simulink library "Backhoe_Lib"  (R2014a)
settings: Solver=ode45  StartTime=0.0  StopTime=10.0  RelTol=1e-3
undefined symbols (not defined in the file): cylinderGray, gcbh, pistonGray, rhoSteel, simmechanics, X, Y, Z
libraries: sm_lib x40, Backhoe_Lib x7, fl_lib x7, nesl_utility x2
(part 2 of 2)

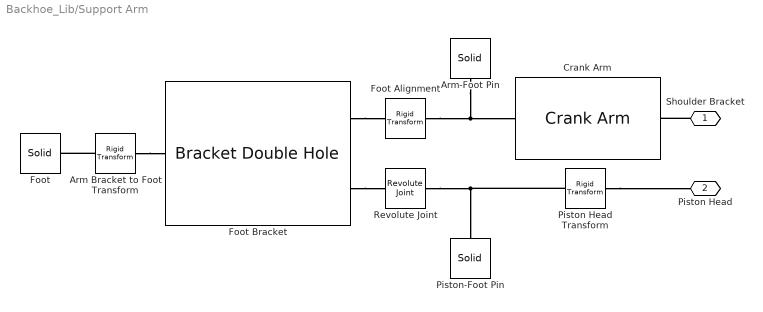
== system Backhoe_Lib/Support Arm ==
  Arm Bracket to Foot Transform : sm_lib/Frames and  Transforms/Rigid  Transform  TranslationMethod=StandardAxis  TranslationLengthUnit=m  TranslationStandardAxis=-Z  TranslationStandardOffset=Tfoot/2  TranslationCartesianOffset=[-Dconn/2 0 -Tfoot/2]  TranslationROffset=0  TranslationROffsetUnits=m  TranslationZOffset=0  TranslationZOffsetUnits=m  TranslationThetaOffset=0  TranslationThetaOffsetUnits=deg  RotationMethod=None  RotationAngleUnits=deg  RotationStandardAxis=-Z  RotationAngle=45  RotationArbitraryAxis=[0 0 1]  FollAlignAxisA=+X  BaseAlignAxisA=+Y  FollAlignAxisB=+Y  BaseAlignAxisB=+Z  BlockFunction=simmechanics.library.frames_transforms.rigid_transform
  Arm-Foot Pin : sm_lib/Body Elements/Solid  InertiaType=CalculateFromGeometry  Mass=1  MassUnits=kg  CenterOfMass=[0 0 0]  CenterOfMassUnits=m  MomentsOfInertia=[1 1 1]  MomentsOfInertiaUnits=kg*m^2  ProductsOfInertia=[0 0 0]  ProductsOfInertiaUnits=kg*m^2  DensityBased=on  Density=rho  DensityUnits=kg/(m^3)  GraphicType=FromGeometry  MarkerShape=Sphere  MarkerSize=10  MarkerSizeUnits=m  GraphicVisPropType=SimpleVisualProperties  GraphicDiffuseColor=pinColor  GraphicSpecularColor=[0.5 0.5 0.5 1.0]  GraphicAmbientColor=[0.15 0.15 0.15 1.0]  GraphicEmissiveColor=[0.0 0.0 0.0 1.0]  GraphicShininess=75  GraphicOpacity=1.0  GeometryShape=Cylinder  RectangleSize=[1 1]  RectangleSizeUnits=m  BrickDimensions=[1 1 1]  BrickDimensionUnits=m  CylinderRadius=Rhole  CylinderRadiusUnits=m  CylinderLength=Lpin  CylinderLengthUnits=m  SphereRadius=1  SphereRadiusUnits=m  EllipsoidRadii=[1 1 1]  EllipsoidRadiiUnits=m  ExtrusionCrossSection=[1 1; 1 1]  ExtrusionCrossSectionUnits=m  ExtrusionLength=Lpin  ExtrusionLengthUnits=m  PolygonNumSides=3  PolygonOuterRadius=1  PolygonOuterRadiusUnits=m  ExtGeomFileUnits=m  RevolutionCrossSection=[1 1; 1 -1; 2 -1; 2 1]  RevolutionCrossSectionUnits=m  RevolutionExtent=Full  RevolutionAngle=180  RevolutionAngleUnits=deg  BlockFunction=simmechanics.library.body_elements.solid
  Crank Arm : Backhoe_Lib/Crank Arm  L=Larm  W=Warm  T=Tarm  D=Dhole  R=Rhole  Nc=25  color=armColor  rho=rho
  Foot : sm_lib/Body Elements/Solid  InertiaType=CalculateFromGeometry  Mass=1  MassUnits=kg  CenterOfMass=[0 0 0]  CenterOfMassUnits=m  MomentsOfInertia=[1 1 1]  MomentsOfInertiaUnits=kg*m^2  ProductsOfInertia=[0 0 0]  ProductsOfInertiaUnits=kg*m^2  DensityBased=on  Density=rho  DensityUnits=kg/(m^3)  GraphicType=FromGeometry  MarkerShape=Sphere  MarkerSize=10  MarkerSizeUnits=m  GraphicVisPropType=SimpleVisualProperties  GraphicDiffuseColor=footColor  GraphicSpecularColor=[0.5 0.5 0.5 1.0]  GraphicAmbientColor=[0.15 0.15 0.15 1.0]  GraphicEmissiveColor=[0.0 0.0 0.0 1.0]  GraphicShininess=75  GraphicOpacity=1.0  GeometryShape=Brick  RectangleSize=[1 1]  RectangleSizeUnits=m  BrickDimensions=[Lfoot Wfoot Tfoot]  BrickDimensionUnits=m  CylinderRadius=1  CylinderRadiusUnits=m  CylinderLength=1  CylinderLengthUnits=m  SphereRadius=1  SphereRadiusUnits=m  EllipsoidRadii=[1 1 1]  EllipsoidRadiiUnits=m  ExtrusionCrossSection=[0 1;1 0; 1 1]  ExtrusionCrossSectionUnits=m  ExtrusionLength=1  ExtrusionLengthUnits=m  PolygonNumSides=3  PolygonOuterRadius=1  PolygonOuterRadiusUnits=m  ExtGeomFileUnits=m  RevolutionCrossSection=[1 1; 1 -1; 2 -1; 2 1]  RevolutionCrossSectionUnits=m  RevolutionExtent=Full  RevolutionAngle=180  RevolutionAngleUnits=deg  BlockFunction=simmechanics.library.body_elements.solid
  Foot Alignment : sm_lib/Frames and  Transforms/Rigid  Transform  TranslationMethod=None  TranslationLengthUnit=m  TranslationStandardAxis=+Z  TranslationStandardOffset=0  TranslationCartesianOffset=[0 0 0]  TranslationROffset=0  TranslationROffsetUnits=m  TranslationZOffset=0  TranslationZOffsetUnits=m  TranslationThetaOffset=0  TranslationThetaOffsetUnits=deg  RotationMethod=StandardAxis  RotationAngleUnits=deg  RotationStandardAxis=+Z  RotationAngle=initAngle  RotationArbitraryAxis=[0 0 1]  FollAlignAxisA=+X  BaseAlignAxisA=+Y  FollAlignAxisB=+Y  BaseAlignAxisB=+Z  BlockFunction=simmechanics.library.frames_transforms.rigid_transform
  Foot Bracket : Backhoe_Lib/Bracket Double Hole  Hbracket=Hhole + Rfillet  Wbracket=Dconn + Rfillet  Tbracket=Tfoot  Dbracket=Wfoot*0.75  Hhole=Hhole  Dhole=Dconn  Rhole=Rhole  Rfillet=Rfillet  Nc=25  bracketColor=bracketColor  rho=rho
  Piston Head Transform : sm_lib/Frames and Transforms/Rigid Transform  TranslationMethod=None  TranslationLengthUnit=m  TranslationStandardAxis=+Z  TranslationStandardOffset=0  TranslationCartesianOffset=[0 0 0]  TranslationROffset=0  TranslationROffsetUnits=m  TranslationZOffset=0  TranslationZOffsetUnits=m  TranslationThetaOffset=0  TranslationThetaOffsetUnits=deg  RotationMethod=AlignedAxes  RotationAngleUnits=deg  RotationStandardAxis=+Z  RotationAngle=0  RotationArbitraryAxis=[0 0 1]  FollAlignAxisA=+Z  BaseAlignAxisA=-Z  FollAlignAxisB=+Y  BaseAlignAxisB=-Y  BlockFunction=simmechanics.library.frames_transforms.rigid_transform
  Piston-Foot Pin : sm_lib/Body Elements/Solid  InertiaType=CalculateFromGeometry  Mass=1  MassUnits=kg  CenterOfMass=[0 0 0]  CenterOfMassUnits=m  MomentsOfInertia=[1 1 1]  MomentsOfInertiaUnits=kg*m^2  ProductsOfInertia=[0 0 0]  ProductsOfInertiaUnits=kg*m^2  DensityBased=on  Density=rho  DensityUnits=kg/(m^3)  GraphicType=FromGeometry  MarkerShape=Sphere  MarkerSize=10  MarkerSizeUnits=m  GraphicVisPropType=SimpleVisualProperties  GraphicDiffuseColor=pinColor  GraphicSpecularColor=[0.5 0.5 0.5 1.0]  GraphicAmbientColor=[0.15 0.15 0.15 1.0]  GraphicEmissiveColor=[0.0 0.0 0.0 1.0]  GraphicShininess=75  GraphicOpacity=1.0  GeometryShape=Cylinder  RectangleSize=[1 1]  RectangleSizeUnits=m  BrickDimensions=[1 1 1]  BrickDimensionUnits=m  CylinderRadius=Rhole  CylinderRadiusUnits=m  CylinderLength=Lpin  CylinderLengthUnits=m  SphereRadius=1  SphereRadiusUnits=m  EllipsoidRadii=[1 1 1]  EllipsoidRadiiUnits=m  ExtrusionCrossSection=[1 1; 1 1]  ExtrusionCrossSectionUnits=m  ExtrusionLength=Lpin  ExtrusionLengthUnits=m  PolygonNumSides=3  PolygonOuterRadius=1  PolygonOuterRadiusUnits=m  ExtGeomFileUnits=m  RevolutionCrossSection=[1 1; 1 -1; 2 -1; 2 1]  RevolutionCrossSectionUnits=m  RevolutionExtent=Full  RevolutionAngle=180  RevolutionAngleUnits=deg  BlockFunction=simmechanics.library.body_elements.solid
  Revolute Joint : sm_lib/Joints/Revolute Joint  SenseConstraintForceX=off  SenseConstraintForceY=off  SenseConstraintForceZ=off  SenseConstraintTorqueX=off  SenseConstraintTorqueY=off  SenseConstraintTorqueZ=off  ConstraintWrenchDir=FollowerOnBase  ConstraintWrenchFrame=BaseFrame  EquilibriumPosition=0  EquilibriumPositionUnits=deg  SpringStiffness=0  SpringStiffnessUnits=N*m/deg  DampingCoefficient=0  DampingCoefficientUnits=N*m/(deg/s)  ActuationMode=NoActuation  SensePosition=off  SenseVelocity=off  SenseAcceleration=off  SenseTorqueForce=off  PositionTargetValue=0  PositionTargetValueUnits=deg  PositionTargetSpecify=off  PositionTargetPriority=High  VelocityTargetValue=0  VelocityTargetValueUnits=deg/s  VelocityTargetSpecify=off  VelocityTargetPriority=High  BlockFunction=simmechanics.library.joints.revolute_joint
  Shoulder Bracket : PMIOPort  Port=1  Side=Right
  Piston Head : PMIOPort  Port=2  Side=Left
  connections:
  Shoulder Bracket/RConn1 -- Crank Arm/RConn1
  Revolute Joint/RConn1 -- Piston Head Transform/LConn1 -- Piston-Foot Pin/RConn1
  Arm Bracket to Foot Transform/RConn1 -- Foot/RConn1
  Arm-Foot Pin/RConn1 -- Crank Arm/LConn1 -- Foot Alignment/RConn1
  Foot Bracket/RConn2 -- Revolute Joint/LConn1
  Foot Bracket/RConn1 -- Foot Alignment/LConn1
  Arm Bracket to Foot Transform/LConn1 -- Foot Bracket/LConn1
  Piston Head Transform/RConn1 -- Piston Head/RConn1

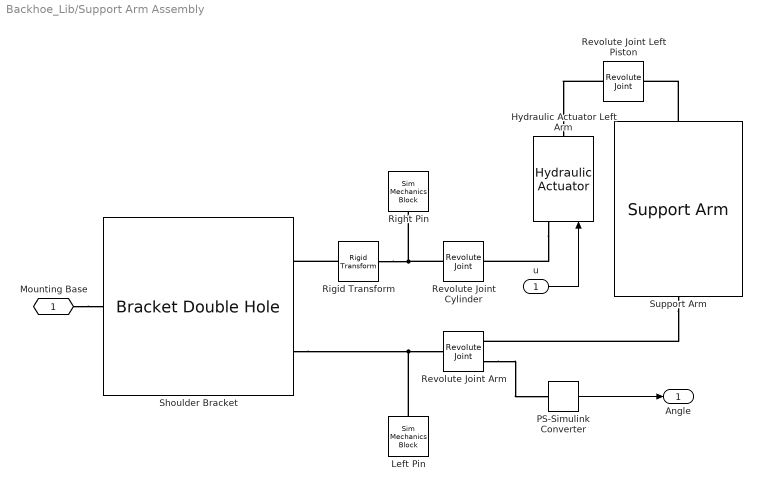
== system Backhoe_Lib/Support Arm Assembly ==
  u : Inport
  Hydraulic Actuator Left Arm : Backhoe_Lib/Hydraulic Actuator  Lcyl=1.35  Rcyl=0.2  Lpist=1.35  Rpist=0.1  Lbase=0.65  Wbase=0.425  Rbp=0.075  Lbp=0.8  Whead=0.275  Lhead=0.5  Rhp=0.075  Lhp=0.9  circlePoints=25  cylColor=cylinderGray  rhoCyl=rho  pistColor=pistonGray  rhoPist=rho  connColor=pinColor  rhoConn=rho
  Left Pin : SimMechanicsBlock  LoadFcn=simmechanics.sli.internal.rtm_callback('LoadFcn',gcbh)  StartFcn=simmechanics.sli.internal.model_callback(bdroot(gcbh),'start');  StopFcn=simmechanics.sli.internal.model_callback(bdroot(gcbh),'stop');  mask(Solid){ClassName=Solid, InertiaType=CalculateFromGeometry, Mass=1, MassUnits=kg, CenterOfMass=[0 0 0], CenterOfMassUnits=m, MomentsOfInertia=[1 1 1], MomentsOfInertiaUnits=kg*m^2, ProductsOfInertia=[0 0 0], ProductsOfInertiaUnits=kg*m^2, DensityBased=on, Density=rho, DensityUnits=kg/(m^3), GraphicType=FromGeometry, MarkerShape=Sphere, MarkerSize=10, MarkerSizeUnits=m, GraphicVisPropType=SimpleVisualProperties, GraphicDiffuseColor=pinColor, GraphicSpecularColor=[0.5 0.5 0.5 1.0], GraphicAmbientColor=[0.15 0.15 0.15 1.0], GraphicEmissiveColor=[0.0 0.0 0.0 1.0], GraphicShininess=75, GraphicOpacity=1.0, GeometryShape=Cylinder, RectangleSize=[1 1], RectangleSizeUnits=m, BrickDimensions=[1 1 1], BrickDimensionUnits=m, CylinderRadius=Rhole, CylinderRadiusUnits=m, CylinderLength=Lpin, CylinderLengthUnits=m, SphereRadius=1, SphereRadiusUnits=m, EllipsoidRadii=[1 1 1], EllipsoidRadiiUnits=m, ExtrusionCrossSection=[1 1; 1 1], ExtrusionCrossSectionUnits=m, ExtrusionLength=1, ExtrusionLengthUnits=m, PolygonNumSides=3, PolygonOuterRadius=1, PolygonOuterRadiusUnits=m, ExtGeomFileName=, ExtGeomFileUnits=m, RevolutionCrossSection=[1 1; 1 -1; 2 -1; 2 1], RevolutionCrossSectionUnits=m, RevolutionExtent=Full, RevolutionAngle=180, RevolutionAngleUnits=deg, BlockFunction=simmechanics.library.body_elements.solid}
      mask prompts: BlockFunction "Block Function"
      settings: PreSaveFcn=simmechanics.sli.internal.rtm_callback('PreSaveFcn',gcbh)  PauseFcn=simmechanics.sli.internal.model_callback(bdroot(gcbh),'pause');  PreCopyFcn=simmechanics.sli.internal.rtm_callback('PreCopyFcn',gcbh)  OpenFcn=simmechanics.sli.internal.block_dialog(gcbh,'open');  CloseFcn=simmechanics.sli.internal.block_dialog(gcbh,'close');  PreDeleteFcn=simmechanics.sli.internal.rtm_callback('PreDeleteFcn',gcbh)
      settings: CopyFcn=|
      | simmechanics.sli.internal.block_dialog(gcbh,'close');
      | simmechanics.sli.internal.rtm_callback('CopyFcn',gcbh)
      settings: DeleteFcn=|
      | simmechanics.sli.internal.block_dialog(gcbh,'close');
      | simmechanics.sli.internal.rtm_callback('DeleteFcn',gcbh)
      settings: ModelCloseFcn=|
      | simmechanics.sli.internal.model_editor_callback(bdroot(gcbh),'close');
      | simmechanics.sli.internal.rtm_callback('ModelCloseFcn',gcbh)
      | simmechanics.sli.internal.model_callback(bdroot(gcbh),'close');
      settings: PostSaveFcn=|
      | simmechanics.sli.internal.model_editor_callback(bdroot(gcbh),'save');
      | simmechanics.sli.internal.rtm_callback('PostSaveFcn',gcbh)
      mask Help: web(simmechanics.sli.internal.block_help(gcbh))
      mask Display: plot([0;1;1;0;0],[0;0;1;1;0]);
  PS-Simulink Converter : nesl_utility/PS-Simulink Converter  PhysicalDomain=network_engine_domain  LeftPortType=input  RightPortType=output  SubClassName=ps_output  PseudoPeriodic=off  Frequencies=[]  Unit=deg  AffineConversion=off
  Revolute Joint Arm : sm_lib/Joints/Revolute Joint  SenseConstraintForceX=off  SenseConstraintForceY=off  SenseConstraintForceZ=off  SenseConstraintTorqueX=off  SenseConstraintTorqueY=off  SenseConstraintTorqueZ=off  ConstraintWrenchDir=FollowerOnBase  ConstraintWrenchFrame=BaseFrame  EquilibriumPosition=0  EquilibriumPositionUnits=deg  SpringStiffness=0  SpringStiffnessUnits=N*m/deg  DampingCoefficient=0  DampingCoefficientUnits=N*m/(deg/s)  ActuationMode=NoActuation  SensePosition=on  SenseVelocity=off  SenseAcceleration=off  SenseTorqueForce=off  PositionTargetValue=-90  PositionTargetValueUnits=deg  PositionTargetSpecify=on  PositionTargetPriority=High  VelocityTargetValue=0  VelocityTargetValueUnits=deg/s  VelocityTargetSpecify=off  VelocityTargetPriority=High  BlockFunction=simmechanics.library.joints.revolute_joint
  Revolute Joint Cylinder : sm_lib/Joints/Revolute Joint  SenseConstraintForceX=off  SenseConstraintForceY=off  SenseConstraintForceZ=off  SenseConstraintTorqueX=off  SenseConstraintTorqueY=off  SenseConstraintTorqueZ=off  ConstraintWrenchDir=FollowerOnBase  ConstraintWrenchFrame=BaseFrame  EquilibriumPosition=0  EquilibriumPositionUnits=deg  SpringStiffness=0  SpringStiffnessUnits=N*m/deg  DampingCoefficient=0  DampingCoefficientUnits=N*m/(deg/s)  ActuationMode=NoActuation  SensePosition=off  SenseVelocity=off  SenseAcceleration=off  SenseTorqueForce=off  PositionTargetValue=0  PositionTargetValueUnits=deg  PositionTargetSpecify=off  PositionTargetPriority=High  VelocityTargetValue=0  VelocityTargetValueUnits=deg/s  VelocityTargetSpecify=off  VelocityTargetPriority=High  BlockFunction=simmechanics.library.joints.revolute_joint
  Revolute Joint Left Piston : sm_lib/Joints/Revolute Joint  SenseConstraintForceX=off  SenseConstraintForceY=off  SenseConstraintForceZ=off  SenseConstraintTorqueX=off  SenseConstraintTorqueY=off  SenseConstraintTorqueZ=off  ConstraintWrenchDir=FollowerOnBase  ConstraintWrenchFrame=BaseFrame  EquilibriumPosition=0  EquilibriumPositionUnits=deg  SpringStiffness=0  SpringStiffnessUnits=N*m/deg  DampingCoefficient=0  DampingCoefficientUnits=N*m/(deg/s)  ActuationMode=NoActuation  SensePosition=off  SenseVelocity=off  SenseAcceleration=off  SenseTorqueForce=off  PositionTargetValue=0  PositionTargetValueUnits=deg  PositionTargetSpecify=off  PositionTargetPriority=High  VelocityTargetValue=0  VelocityTargetValueUnits=deg/s  VelocityTargetSpecify=off  VelocityTargetPriority=High  BlockFunction=simmechanics.library.joints.revolute_joint
  Right Pin : SimMechanicsBlock  LoadFcn=simmechanics.sli.internal.rtm_callback('LoadFcn',gcbh)  StartFcn=simmechanics.sli.internal.model_callback(bdroot(gcbh),'start');  StopFcn=simmechanics.sli.internal.model_callback(bdroot(gcbh),'stop');  mask(Solid){ClassName=Solid, InertiaType=CalculateFromGeometry, Mass=1, MassUnits=kg, CenterOfMass=[0 0 0], CenterOfMassUnits=m, MomentsOfInertia=[1 1 1], MomentsOfInertiaUnits=kg*m^2, ProductsOfInertia=[0 0 0], ProductsOfInertiaUnits=kg*m^2, DensityBased=on, Density=rho, DensityUnits=kg/(m^3), GraphicType=FromGeometry, MarkerShape=Sphere, MarkerSize=10, MarkerSizeUnits=m, GraphicVisPropType=SimpleVisualProperties, GraphicDiffuseColor=pinColor, GraphicSpecularColor=[0.5 0.5 0.5 1.0], GraphicAmbientColor=[0.15 0.15 0.15 1.0], GraphicEmissiveColor=[0.0 0.0 0.0 1.0], GraphicShininess=75, GraphicOpacity=1.0, GeometryShape=Cylinder, RectangleSize=[1 1], RectangleSizeUnits=m, BrickDimensions=[1 1 1], BrickDimensionUnits=m, CylinderRadius=Rhole, CylinderRadiusUnits=m, CylinderLength=Lpin, CylinderLengthUnits=m, SphereRadius=1, SphereRadiusUnits=m, EllipsoidRadii=[1 1 1], EllipsoidRadiiUnits=m, ExtrusionCrossSection=[1 1; 1 1], ExtrusionCrossSectionUnits=m, ExtrusionLength=1, ExtrusionLengthUnits=m, PolygonNumSides=3, PolygonOuterRadius=1, PolygonOuterRadiusUnits=m, ExtGeomFileName=, ExtGeomFileUnits=m, RevolutionCrossSection=[1 1; 1 -1; 2 -1; 2 1], RevolutionCrossSectionUnits=m, RevolutionExtent=Full, RevolutionAngle=180, RevolutionAngleUnits=deg, BlockFunction=simmechanics.library.body_elements.solid}
      mask prompts: BlockFunction "Block Function"
      settings: PreSaveFcn=simmechanics.sli.internal.rtm_callback('PreSaveFcn',gcbh)  PauseFcn=simmechanics.sli.internal.model_callback(bdroot(gcbh),'pause');  PreCopyFcn=simmechanics.sli.internal.rtm_callback('PreCopyFcn',gcbh)  OpenFcn=simmechanics.sli.internal.block_dialog(gcbh,'open');  CloseFcn=simmechanics.sli.internal.block_dialog(gcbh,'close');  PreDeleteFcn=simmechanics.sli.internal.rtm_callback('PreDeleteFcn',gcbh)
      settings: CopyFcn=|
      | simmechanics.sli.internal.block_dialog(gcbh,'close');
      | simmechanics.sli.internal.rtm_callback('CopyFcn',gcbh)
      settings: DeleteFcn=|
      | simmechanics.sli.internal.block_dialog(gcbh,'close');
      | simmechanics.sli.internal.rtm_callback('DeleteFcn',gcbh)
      settings: ModelCloseFcn=|
      | simmechanics.sli.internal.model_editor_callback(bdroot(gcbh),'close');
      | simmechanics.sli.internal.rtm_callback('ModelCloseFcn',gcbh)
      | simmechanics.sli.internal.model_callback(bdroot(gcbh),'close');
      settings: PostSaveFcn=|
      | simmechanics.sli.internal.model_editor_callback(bdroot(gcbh),'save');
      | simmechanics.sli.internal.rtm_callback('PostSaveFcn',gcbh)
      mask Help: web(simmechanics.sli.internal.block_help(gcbh))
      mask Display: plot([0;1;1;0;0],[0;0;1;1;0]);
  Rigid Transform : sm_lib/Frames and  Transforms/Rigid  Transform  TranslationMethod=None  TranslationLengthUnit=m  TranslationStandardAxis=+Z  TranslationStandardOffset=0  TranslationCartesianOffset=[0 0 0]  TranslationROffset=0  TranslationROffsetUnits=m  TranslationZOffset=0  TranslationZOffsetUnits=m  TranslationThetaOffset=0  TranslationThetaOffsetUnits=deg  RotationMethod=AlignedAxes  RotationAngleUnits=deg  RotationStandardAxis=+Z  RotationAngle=0  RotationArbitraryAxis=[0 0 1]  FollAlignAxisA=+Z  BaseAlignAxisA=-Z  FollAlignAxisB=+Y  BaseAlignAxisB=-Y  BlockFunction=simmechanics.library.frames_transforms.rigid_transform
  Shoulder Bracket : Backhoe_Lib/Bracket Double Hole  Hbracket=Hbracket  Wbracket=Wbracket  Tbracket=Tbracket  Dbracket=Dbracket  Hhole=HShoulderHole  Dhole=DShoulderHole  Rhole=RShoulderHole  Rfillet=RShoulderFillet  Nc=25  bracketColor=shoulderColor  rho=rho
  Support Arm : Backhoe_Lib/Support Arm  Larm=Larm  Warm=Warm  Tarm=Tarm  Dhole=Dhole  Rhole=Rhole  initAngle=AFAngle  Lfoot=Lfoot  Wfoot=Wfoot  Tfoot=Tfoot  Dconn=Dconn  Hhole=Hhole  Rfillet=Rfillet  Lpin=Lpin  circlePoints=circlePoints  armColor=armColor  bracketColor=bracketColor  footColor=footColor  pinColor=pinColor  rho=rho
  Mounting Base : PMIOPort  Port=1  Side=Left
  Angle : Outport
  wires:
  PS-Simulink Converter/1 -> Angle/1
  u/1 -> Hydraulic Actuator Left Arm/1
  connections:
  Support Arm/LConn1 -- Revolute Joint Left Piston/LConn1
  Revolute Joint Arm/RConn2 -- PS-Simulink Converter/LConn1
  Support Arm/RConn1 -- Revolute Joint Arm/RConn1
  Revolute Joint Cylinder/LConn1 -- Rigid Transform/RConn1 -- Right Pin/RConn1
  Shoulder Bracket/RConn2 -- Revolute Joint Arm/LConn1 -- Left Pin/RConn1
  Mounting Base/RConn1 -- Shoulder Bracket/LConn1
  Revolute Joint Left Piston/RConn1 -- Hydraulic Actuator Left Arm/RConn1
  Hydraulic Actuator Left Arm/LConn1 -- Revolute Joint Cylinder/RConn1
  Rigid Transform/LConn1 -- Shoulder Bracket/RConn1

== system Backhoe_Lib/Wheel ==
  Rim : SimMechanicsBlock  LoadFcn=simmechanics.sli.internal.rtm_callback('LoadFcn',gcbh)  StartFcn=simmechanics.sli.internal.model_callback(bdroot(gcbh),'start');  StopFcn=simmechanics.sli.internal.model_callback(bdroot(gcbh),'stop');  mask(Solid){ClassName=Solid, InertiaType=CalculateFromGeometry, Mass=1, MassUnits=kg, CenterOfMass=[0 0 0], CenterOfMassUnits=m, MomentsOfInertia=[1 1 1], MomentsOfInertiaUnits=kg*m^2, ProductsOfInertia=[0 0 0], ProductsOfInertiaUnits=kg*m^2, DensityBased=on, Density=rhoWheel, DensityUnits=kg/(m^3), GraphicType=FromGeometry, MarkerShape=Sphere, MarkerSize=10, MarkerSizeUnits=m, GraphicVisPropType=SimpleVisualProperties, GraphicDiffuseColor=wheelColor, GraphicSpecularColor=[0.5 0.5 0.5 1.0], GraphicAmbientColor=[0.15 0.15 0.15 1.0], GraphicEmissiveColor=[0.0 0.0 0.0 1.0], GraphicShininess=75, GraphicOpacity=1.0, GeometryShape=GeneralSolidOfRevolution, RectangleSize=[1 1], RectangleSizeUnits=m, BrickDimensions=[1 1 1], BrickDimensionUnits=m, CylinderRadius=1.75, CylinderRadiusUnits=m, CylinderLength=1.5, CylinderLengthUnits=m, SphereRadius=1, SphereRadiusUnits=m, EllipsoidRadii=[1 1 1], EllipsoidRadiiUnits=m, ExtrusionCrossSection=tirePoints, ExtrusionCrossSectionUnits=m, ExtrusionLength=W, ExtrusionLengthUnits=m, PolygonNumSides=3, PolygonOuterRadius=1, PolygonOuterRadiusUnits=m, ExtGeomFileName=, ExtGeomFileUnits=m, RevolutionCrossSection=rimPoints, RevolutionCrossSectionUnits=m, RevolutionExtent=Full, RevolutionAngle=180, RevolutionAngleUnits=deg, BlockFunction=simmechanics.library.body_elements.solid}
      mask prompts: BlockFunction "Block Function"
      settings: PreSaveFcn=simmechanics.sli.internal.rtm_callback('PreSaveFcn',gcbh)  PauseFcn=simmechanics.sli.internal.model_callback(bdroot(gcbh),'pause');  PreCopyFcn=simmechanics.sli.internal.rtm_callback('PreCopyFcn',gcbh)  OpenFcn=simmechanics.sli.internal.block_dialog(gcbh,'open');  CloseFcn=simmechanics.sli.internal.block_dialog(gcbh,'close');  PreDeleteFcn=simmechanics.sli.internal.rtm_callback('PreDeleteFcn',gcbh)
      settings: CopyFcn=|
      | simmechanics.sli.internal.block_dialog(gcbh,'close');
      | simmechanics.sli.internal.rtm_callback('CopyFcn',gcbh)
      settings: DeleteFcn=|
      | simmechanics.sli.internal.block_dialog(gcbh,'close');
      | simmechanics.sli.internal.rtm_callback('DeleteFcn',gcbh)
      settings: ModelCloseFcn=|
      | simmechanics.sli.internal.model_editor_callback(bdroot(gcbh),'close');
      | simmechanics.sli.internal.rtm_callback('ModelCloseFcn',gcbh)
      | simmechanics.sli.internal.model_callback(bdroot(gcbh),'close');
      settings: PostSaveFcn=|
      | simmechanics.sli.internal.model_editor_callback(bdroot(gcbh),'save');
      | simmechanics.sli.internal.rtm_callback('PostSaveFcn',gcbh)
      mask Help: web(simmechanics.sli.internal.block_help(gcbh))
      mask Display: plot([0;1;1;0;0],[0;0;1;1;0]);
  Rim  Transform : sm_lib/Frames and Transforms/Rigid Transform  TranslationMethod=StandardAxis  TranslationLengthUnit=m  TranslationStandardAxis=+Z  TranslationStandardOffset=W*0.85/2  TranslationCartesianOffset=[0 0 0]  TranslationROffset=0  TranslationROffsetUnits=m  TranslationZOffset=0  TranslationZOffsetUnits=m  TranslationThetaOffset=0  TranslationThetaOffsetUnits=deg  RotationMethod=None  RotationAngleUnits=deg  RotationStandardAxis=+Z  RotationAngle=0  RotationArbitraryAxis=[0 0 1]  FollAlignAxisA=+X  BaseAlignAxisA=+Y  FollAlignAxisB=+Y  BaseAlignAxisB=+Z  BlockFunction=simmechanics.library.frames_transforms.rigid_transform
  Tire : sm_lib/Body Elements/Solid  InertiaType=CalculateFromGeometry  Mass=1  MassUnits=kg  CenterOfMass=[0 0 0]  CenterOfMassUnits=m  MomentsOfInertia=[1 1 1]  MomentsOfInertiaUnits=kg*m^2  ProductsOfInertia=[0 0 0]  ProductsOfInertiaUnits=kg*m^2  DensityBased=on  Density=rhoTire  DensityUnits=kg/(m^3)  GraphicType=FromGeometry  MarkerShape=Sphere  MarkerSize=10  MarkerSizeUnits=m  GraphicVisPropType=SimpleVisualProperties  GraphicDiffuseColor=tireColor  GraphicSpecularColor=[0.5 0.5 0.5 1.0]  GraphicAmbientColor=[0.15 0.15 0.15 1.0]  GraphicEmissiveColor=[0.0 0.0 0.0 1.0]  GraphicShininess=75  GraphicOpacity=1.0  GeometryShape=GeneralExtrusion  RectangleSize=[1 1]  RectangleSizeUnits=m  BrickDimensions=[1 1 1]  BrickDimensionUnits=m  CylinderRadius=1.75  CylinderRadiusUnits=m  CylinderLength=1.5  CylinderLengthUnits=m  SphereRadius=1  SphereRadiusUnits=m  EllipsoidRadii=[1 1 1]  EllipsoidRadiiUnits=m  ExtrusionCrossSection=tirePoints  ExtrusionCrossSectionUnits=m  ExtrusionLength=W  ExtrusionLengthUnits=m  PolygonNumSides=3  PolygonOuterRadius=1  PolygonOuterRadiusUnits=m  ExtGeomFileType=STL  ExtGeomFileUnits=m  RevolutionCrossSection=[1 1; 1 -1; 2 -1; 2 1]  RevolutionCrossSectionUnits=m  RevolutionExtent=Full  RevolutionAngle=180  RevolutionAngleUnits=deg  BlockFunction=simmechanics.library.body_elements.solid
  Wheel : sm_lib/Body Elements/Solid  InertiaType=CalculateFromGeometry  Mass=1  MassUnits=kg  CenterOfMass=[0 0 0]  CenterOfMassUnits=m  MomentsOfInertia=[1 1 1]  MomentsOfInertiaUnits=kg*m^2  ProductsOfInertia=[0 0 0]  ProductsOfInertiaUnits=kg*m^2  DensityBased=on  Density=rhoWheel  DensityUnits=kg/(m^3)  GraphicType=FromGeometry  MarkerShape=Sphere  MarkerSize=10  MarkerSizeUnits=m  GraphicVisPropType=SimpleVisualProperties  GraphicDiffuseColor=wheelColor  GraphicSpecularColor=[0.5 0.5 0.5 1.0]  GraphicAmbientColor=[0.15 0.15 0.15 1.0]  GraphicEmissiveColor=[0.0 0.0 0.0 1.0]  GraphicShininess=75  GraphicOpacity=1.0  GeometryShape=GeneralExtrusion  RectangleSize=[1 1]  RectangleSizeUnits=m  BrickDimensions=[1 1 1]  BrickDimensionUnits=m  CylinderRadius=1.75  CylinderRadiusUnits=m  CylinderLength=1.5  CylinderLengthUnits=m  SphereRadius=1  SphereRadiusUnits=m  EllipsoidRadii=[1 1 1]  EllipsoidRadiiUnits=m  ExtrusionCrossSection=wheelPoints  ExtrusionCrossSectionUnits=m  ExtrusionLength=W*0.85  ExtrusionLengthUnits=m  PolygonNumSides=3  PolygonOuterRadius=1  PolygonOuterRadiusUnits=m  ExtGeomFileType=STL  ExtGeomFileUnits=m  RevolutionCrossSection=[1 1; 1 -1; 2 -1; 2 1]  RevolutionCrossSectionUnits=m  RevolutionExtent=Full  RevolutionAngle=180  RevolutionAngleUnits=deg  BlockFunction=simmechanics.library.body_elements.solid
  Axle : PMIOPort  Port=1  Side=Left
  connections:
  Axle/RConn1 -- Tire/RConn1 -- Rim  Transform/LConn1 -- Wheel/RConn1
  Rim  Transform/RConn1 -- Rim/RConn1

== system Backhoe_Lib/Hydraulic Actuator/Cylinder Assembly ==
  Base to Cylinder Transform : sm_lib/Frames and Transforms/Rigid Transform  TranslationMethod=StandardAxis  TranslationLengthUnit=m  TranslationStandardAxis=-Z  TranslationStandardOffset=(Lcyl/2)  TranslationCartesianOffset=[0 0 0]  TranslationROffset=0  TranslationROffsetUnits=m  TranslationZOffset=0  TranslationZOffsetUnits=m  TranslationThetaOffset=0  TranslationThetaOffsetUnits=deg  RotationMethod=AlignedAxes  RotationAngleUnits=deg  RotationStandardAxis=+X  RotationAngle=90  RotationArbitraryAxis=[0 0 1]  FollAlignAxisA=+X  BaseAlignAxisA=+X  FollAlignAxisB=+Z  BaseAlignAxisB=-Z  BlockFunction=simmechanics.library.frames_transforms.rigid_transform
  Cylinder : sm_lib/Body Elements/Solid  InertiaType=CalculateFromGeometry  Mass=1  MassUnits=kg  CenterOfMass=[0 0 0]  CenterOfMassUnits=m  MomentsOfInertia=[1 1 1]  MomentsOfInertiaUnits=kg*m^2  ProductsOfInertia=[0 0 0]  ProductsOfInertiaUnits=kg*m^2  DensityBased=on  Density=rhoCyl  DensityUnits=kg/(m^3)  GraphicType=FromGeometry  MarkerShape=Sphere  MarkerSize=10  MarkerSizeUnits=m  GraphicVisPropType=SimpleVisualProperties  GraphicDiffuseColor=cylColor  GraphicSpecularColor=[0.5 0.5 0.5 1.0]  GraphicAmbientColor=[0.15 0.15 0.15 1.0]  GraphicEmissiveColor=[0.0 0.0 0.0 1.0]  GraphicShininess=75  GraphicOpacity=1.0  GeometryShape=GeneralExtrusion  RectangleSize=[1 1]  RectangleSizeUnits=m  BrickDimensions=[3 0.5 0.5]  BrickDimensionUnits=m  CylinderRadius=Rcyl  CylinderRadiusUnits=m  CylinderLength=Lcyl  CylinderLengthUnits=m  SphereRadius=1  SphereRadiusUnits=m  EllipsoidRadii=[1 1 1]  EllipsoidRadiiUnits=m  ExtrusionCrossSection=cylSection  ExtrusionCrossSectionUnits=m  ExtrusionLength=Lcyl  ExtrusionLengthUnits=m  PolygonNumSides=3  PolygonOuterRadius=1  PolygonOuterRadiusUnits=m  ExtGeomFileType=STL  ExtGeomFileUnits=m  RevolutionCrossSection=[1 1; 1 -1; 2 -1; 2 1]  RevolutionCrossSectionUnits=m  RevolutionExtent=Full  RevolutionAngle=180  RevolutionAngleUnits=deg  BlockFunction=simmechanics.library.body_elements.solid
  Single Bracket : Backhoe_Lib/Single Bracket  Hbracket=Lbase  Wbracket=Wbase  Tbracket=Wbase  Hhole=Lbase-(Wbase/2)  Rhole=Rbp  Nc=25  bracketColor=connColor  rho=rhoConn
  Base Hole : PMIOPort  Port=1  Side=Right
  Prismatic : PMIOPort  Port=2  Side=Left
  connections:
  Prismatic/RConn1 -- Base to Cylinder Transform/LConn1 -- Cylinder/RConn1
  Single Bracket/LConn1 -- Base to Cylinder Transform/RConn1
  Single Bracket/RConn1 -- Base Hole/RConn1

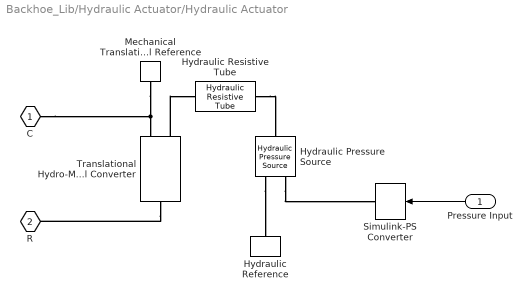
== system Backhoe_Lib/Hydraulic Actuator/Hydraulic Actuator ==
  Pressure Input : Inport
  Hydraulic Pressure Source : fl_lib/Hydraulic/Hydraulic Sources/Hydraulic Pressure Source  q_Log=off  p_Log=off  LocalVarNames=|q|p  LocalVarDescs=|q|p  LocalVarLogging=[0 0]
  Hydraulic Reference : fl_lib/Hydraulic/Hydraulic Elements/Hydraulic Reference  q_Log=off  LocalVarNames=|q  LocalVarDescs=|q  LocalVarLogging=0
  Hydraulic Resistive Tube : fl_lib/Hydraulic/Hydraulic Elements/Hydraulic Resistive Tube  cs_type=1  d_in=0.01 m  area=1e-4 m^2  D_h=0.0112 m  s_factor=64  length=5 m  length_ad=3 m  roughness=2.5e-5 m  Re_lam=2e+3  Re_turb=4e+3  length_eff=6 m  rel_roughness=0.001  f_lam=0.03  f_turb=0.04  f_gain=5e-6  q_Log=off  p_Log=off  power_Log=off  LocalVarNames=|flow_rate|pr_loss|Re|fr_coef|power  LocalVarDescs=|Flow rate through the tube m^3/s)|Pressure loss across the tube (Pa)|Reynolds number|Friction coefficient|Power dissipated in the tube (W)  LocalVarLogging=[0 0 0 0 0]
  Mechanical Translational Reference : fl_lib/Mechanical/Translational Elements/Mechanical Translational Reference
  Simulink-PS Converter : nesl_utility/Simulink-PS Converter  PhysicalDomain=network_engine_domain  LeftPortType=input  RightPortType=output  SubClassName=ps_input  PseudoPeriodic=off  Frequencies=[]  NoiseDistribution=none  NoiseParameters=[]  Unit=Pa  AffineConversion=off  InputFilterTimeConstant=.001  UdotUserProvided=1  SimscapeFilterOrder=1  InputFiltering=off
  Translational Hydro-Mechanical Converter : fl_lib/Hydraulic/Hydraulic Elements/Translational Hydro-Mechanical Converter  area=pi*(Rcyl^2) m^2  or=1  compressibility=0  init_pos=0 m  V_dead=1e-4 m^3  k_sh=1.4  initial_pressure=0 Pa
  C : PMIOPort  Port=1  Side=Right
  R : PMIOPort  Port=2  Side=Right
  wires:
  Pressure Input/1 -> Simulink-PS Converter/1
  connections:
  Translational Hydro-Mechanical Converter/RConn1 -- R/RConn1
  Hydraulic Pressure Source/RConn1 -- Simulink-PS Converter/RConn1
  C/RConn1 -- Mechanical Translational Reference/LConn1 -- Translational Hydro-Mechanical Converter/LConn1
  Hydraulic Pressure Source/RConn2 -- Hydraulic Reference/LConn1
  Translational Hydro-Mechanical Converter/LConn2 -- Hydraulic Resistive Tube/LConn1
  Hydraulic Resistive Tube/RConn1 -- Hydraulic Pressure Source/LConn1

== system Backhoe_Lib/Hydraulic Actuator/Piston Assembly ==
  Piston : sm_lib/Body Elements/Solid  InertiaType=CalculateFromGeometry  Mass=1  MassUnits=kg  CenterOfMass=[0 0 0]  CenterOfMassUnits=m  MomentsOfInertia=[1 1 1]  MomentsOfInertiaUnits=kg*m^2  ProductsOfInertia=[0 0 0]  ProductsOfInertiaUnits=kg*m^2  DensityBased=on  Density=rhoPist  DensityUnits=kg/(m^3)  GraphicType=FromGeometry  MarkerShape=Sphere  MarkerSize=10  MarkerSizeUnits=m  GraphicVisPropType=SimpleVisualProperties  GraphicDiffuseColor=pistColor  GraphicSpecularColor=[0.5 0.5 0.5 1.0]  GraphicAmbientColor=[0.15 0.15 0.15 1.0]  GraphicEmissiveColor=[0.0 0.0 0.0 1.0]  GraphicShininess=75  GraphicOpacity=1.0  GeometryShape=Cylinder  RectangleSize=[1 1]  RectangleSizeUnits=m  BrickDimensions=[3 0.5 0.5]  BrickDimensionUnits=m  CylinderRadius=Rpist  CylinderRadiusUnits=m  CylinderLength=Lpist  CylinderLengthUnits=m  SphereRadius=1  SphereRadiusUnits=m  EllipsoidRadii=[1 1 1]  EllipsoidRadiiUnits=m  ExtrusionCrossSection=[1 1; -1 1; -1 -1; 1 -1]  ExtrusionCrossSectionUnits=m  ExtrusionLength=1  ExtrusionLengthUnits=m  PolygonNumSides=3  PolygonOuterRadius=1  PolygonOuterRadiusUnits=m  ExtGeomFileType=STL  ExtGeomFileUnits=m  RevolutionCrossSection=[1 1; 1 -1; 2 -1; 2 1]  RevolutionCrossSectionUnits=m  RevolutionExtent=Full  RevolutionAngle=180  RevolutionAngleUnits=deg  BlockFunction=simmechanics.library.body_elements.solid
  Piston to Head Transform : sm_lib/Frames and Transforms/Rigid Transform  TranslationMethod=StandardAxis  TranslationLengthUnit=m  TranslationStandardAxis=+Z  TranslationStandardOffset=Lpist/2  TranslationCartesianOffset=[0 0 0]  TranslationROffset=0  TranslationROffsetUnits=m  TranslationZOffset=0  TranslationZOffsetUnits=m  TranslationThetaOffset=0  TranslationThetaOffsetUnits=deg  RotationMethod=AlignedAxes  RotationAngleUnits=deg  RotationStandardAxis=-X  RotationAngle=90  RotationArbitraryAxis=[0 0 1]  FollAlignAxisA=+Y  BaseAlignAxisA=-Y  FollAlignAxisB=+Z  BaseAlignAxisB=+Z  BlockFunction=simmechanics.library.frames_transforms.rigid_transform
  Single Bracket : Backhoe_Lib/Single Bracket  Hbracket=Lbase  Wbracket=Wbase  Tbracket=Whead  Hhole=Lhead-(Whead/2)  Rhole=Rhp  Nc=25  bracketColor=connColor  rho=rhoConn
  Prismatic : PMIOPort  Port=1  Side=Left
  Head Hole : PMIOPort  Port=2  Side=Right
  connections:
  Piston/RConn1 -- Piston to Head Transform/LConn1 -- Prismatic/RConn1
  Piston to Head Transform/RConn1 -- Single Bracket/LConn1
  Single Bracket/RConn1 -- Head Hole/RConn1

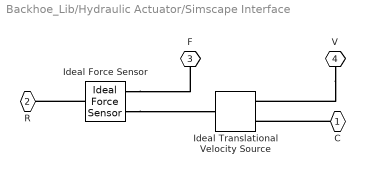
== system Backhoe_Lib/Hydraulic Actuator/Simscape Interface ==
  Ideal Force Sensor : fl_lib/Mechanical/Mechanical Sensors/Ideal Force Sensor
  Ideal Translational Velocity Source : fl_lib/Mechanical/Mechanical Sources/Ideal Translational Velocity Source
  C : PMIOPort  Port=1  Side=Right
  R : PMIOPort  Port=2  Side=Right
  F : PMIOPort  Port=3  Side=Left
  V : PMIOPort  Port=4  Side=Left
  connections:
  Ideal Force Sensor/RConn1 -- Ideal Translational Velocity Source/LConn1
  V/RConn1 -- Ideal Translational Velocity Source/RConn1
  C/RConn1 -- Ideal Translational Velocity Source/RConn2
  Ideal Force Sensor/LConn1 -- R/RConn1
  Ideal Force Sensor/RConn2 -- F/RConn1
